simulink model "Wind"  (R2024b)
settings: Solver=ode23t  StartTime=0.0  StopTime=120  RelTol=1e-3
settings Model: Creator=Ioannis Vourkas  LastModifiedBy=HP

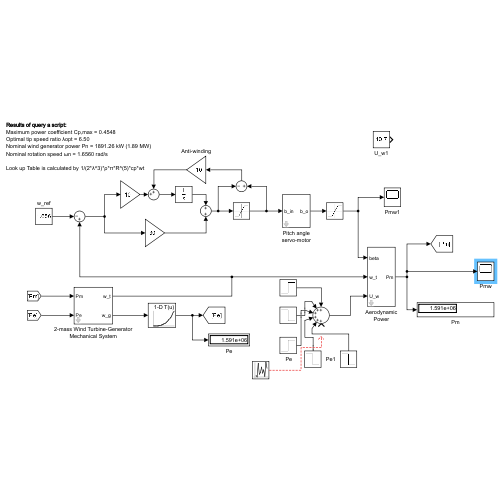
[thumbnail: Simulink's stored preview of the top-level diagram]
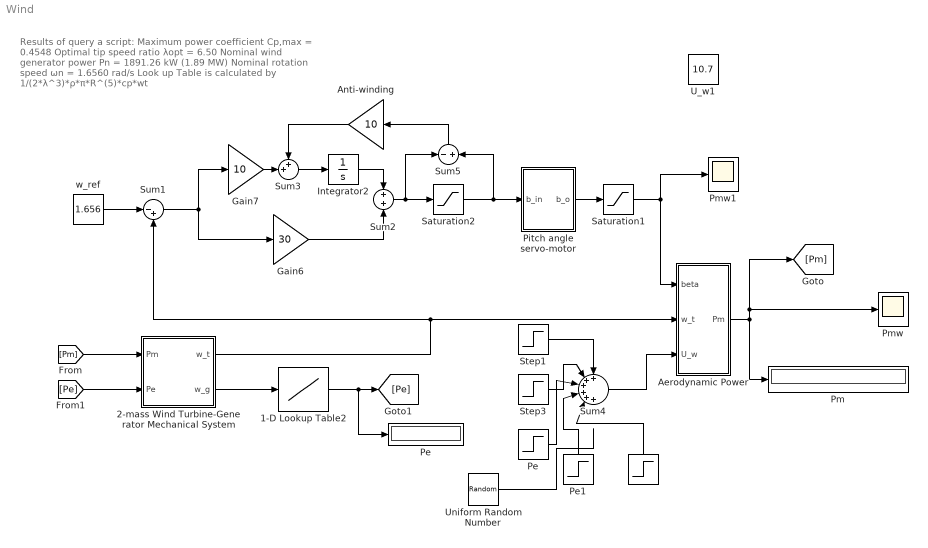
== system Wind ==
  note: Results of query a script:
      | Maximum power coefficient Cp,max = 0.4548
      | Optimal tip speed ratio λopt = 6.50
      | Nominal wind generator power Pn = 1891.26 kW (1.89 MW)
      | Nominal rotation speed ωn = 1.6560 rad/s
      |
      | Look up Table is calculated by 1/(2*λ^3)*ρ*π*R^(5)*cp*wt
  " " : Step  Time=35  After=-0.2  SampleTime=0
  " Pe" : Step  Time=20  After=0.45  SampleTime=0
  " Pe1" : Step  Time=25  After=-0.65  SampleTime=0
  1-D Lookup Table2 : Lookup_n-D  NumberOfTableDimensions=1  BreakpointsForDimension1=[0:0.05:1.656]  Table=416.257e3*[0:0.05:1.656].^3  InternalRulePriority=Speed  RndMeth=Simplest
  2-mass Wind Turbine-Generator Mechanical System : Subsystem  mask{K=15e6, D=5e6, Jt=8e6, Jn=100, w_init=1.65, w_inig=1.65}
      mask prompts: K "Elasticity"; D "Damping"; Jt "Turb Moment of Inertia"; Jn "Gen Moment of Inertia"; w_init "Initial turb w"; w_inig "Initial gen w"
  Aerodynamic Power : Subsystem  mask{R=42, ro=1.225, z=[0.0045, 0.0290], c=[0.22, 116.00, 0.20, 0.00, 5.00, 12.20]}
      mask prompts: R "Radius"; ro "Air density"; z "Z parameters"; c "C parameters"
  Anti-winding : Gain  Gain=10
  Gain6 : Gain  Gain=30
  Gain7 : Gain  Gain=10
  Integrator2 : Integrator
  Pe : Display
  Pitch angle servo-motor : Subsystem  mask{Tpam=0.2}
      mask prompts: Tpam "Pitch angle motor"
  Pm : Display
  Pmw : Scope
  Pmw1 : Scope
  Saturation1 : Saturate  UpperLimit=90  LowerLimit=0
  Saturation2 : Saturate  UpperLimit=90  LowerLimit=0
  Step1 : Step  Time=7  Before=10.7  After=11  SampleTime=0
  Step3 : Step  Time=13  Before=0.10  After=-0.5  SampleTime=0
  Sum1 : Sum  Inputs=|-+
  Sum2 : Sum  Inputs=+|+
  Sum3 : Sum  Inputs=++|
  Sum4 : Sum  Inputs=++++++
  Sum5 : Sum  Inputs=-|+
  U_w1 : Constant  Value=10.7
  Uniform Random Number : UniformRandomNumber  Minimum=1.3  Maximum=3.3  SampleTime=0.1
  w_ref : Constant  Value=1.656
  wires:
  Gain6/1 -> Sum2/2
  Integrator2/1 -> Sum2/1
  Gain7/1 -> Sum3/2
  Saturation1/1 -> Aerodynamic Power/1(beta), Pmw1/1
  Sum5/1 -> Anti-winding/1
  Anti-winding/1 -> Sum3/1
  Sum3/1 -> Integrator2/1
  Saturation2/1 -> Pitch angle servo-motor/1(b_in), Sum5/2
  Pitch angle servo-motor/1(b_o) -> Saturation1/1
  Sum2/1 -> Saturation2/1, Sum5/1
  Sum1/1 -> Gain6/1, Gain7/1
  w_ref/1 -> Sum1/1
  2-mass Wind Turbine-Generator Mechanical System/2(w_g) -> 1-D Lookup Table2/1
  2-mass Wind Turbine-Generator Mechanical System/1(w_t) -> Sum1/2, Aerodynamic Power/2(w_t)
  [Pe] -> 2-mass Wind Turbine-Generator Mechanical System/2(Pe)
  [Pm] -> 2-mass Wind Turbine-Generator Mechanical System/1(Pm)
  1-D Lookup Table2/1 -> Pe/1, [Pe]
  Aerodynamic Power/1(Pm) -> Pmw/1, [Pm], Pm/1
  Step3/1 -> Sum4/2
  " Pe"/1 -> Sum4/3
  Step1/1 -> Sum4/1
  " Pe1"/1 -> Sum4/4
  " "/1 -> Sum4/5
  Sum4/1 -> Aerodynamic Power/3(U_w)
  Uniform Random Number/1 -> ?

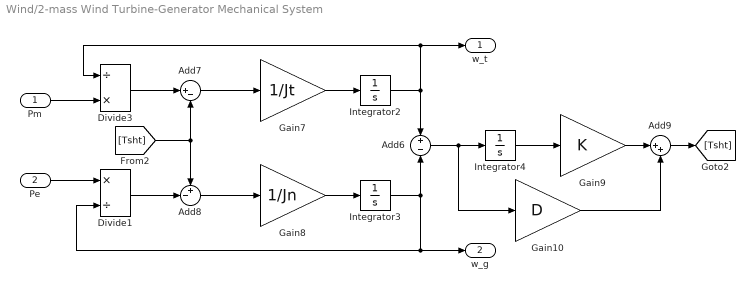
== system Wind/2-mass Wind Turbine-Generator Mechanical System ==
  Pm : Inport
  Pe : Inport  Port=2
  Add6 : Sum  Inputs=+|-
  Add7 : Sum  Inputs=|+-
  Add8 : Sum  Inputs=+-|
  Add9 : Sum  Inputs=|++
  Divide1 : Product  Inputs=*/
  Divide3 : Product  Inputs=/*
  Gain10 : Gain  Gain=D
  Gain7 : Gain  Gain=1/Jt
  Gain8 : Gain  Gain=1/Jn
  Gain9 : Gain  Gain=K
  Integrator2 : Integrator  InitialCondition=w_init
  Integrator3 : Integrator  InitialCondition=w_inig
  Integrator4 : Integrator  InitialCondition=0.35
  w_t : Outport
  w_g : Outport  Port=2
  wires:
  Pm/1 -> Divide3/2
  Pe/1 -> Divide1/1
  Add7/1 -> Gain7/1
  Add8/1 -> Gain8/1
  Gain9/1 -> Add9/1
  Divide3/1 -> Add7/1
  [Tsht] -> Add7/2, Add8/1
  Gain10/1 -> Add9/2
  Divide1/1 -> Add8/2
  Integrator4/1 -> Gain9/1
  Integrator3/1 -> Add6/2, w_g/1, Divide1/2
  Add6/1 -> Integrator4/1, Gain10/1
  Gain7/1 -> Integrator2/1
  Integrator2/1 -> w_t/1, Divide3/1, Add6/1
  Gain8/1 -> Integrator3/1
  Add9/1 -> [Tsht]

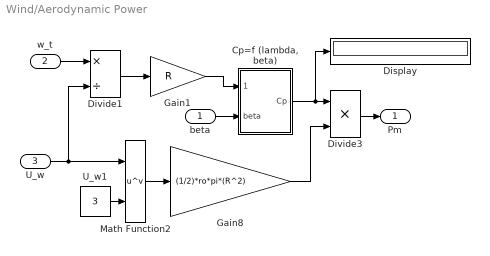
== system Wind/Aerodynamic Power ==
  beta : Inport
  w_t : Inport  Port=2
  U_w : Inport  Port=3
  "Cp=f (lambda, beta)" : Subsystem
  Display : Display
  Divide1 : Product  Inputs=*/
  Divide3 : Product  Inputs=**
  Gain1 : Gain  Gain=R
  Gain8 : Gain  Gain=(1/2)*ro*pi*(R^2)
  Math Function2 : Math  Operator=pow
  U_w1 : Constant  Value=3
  Pm : Outport
  wires:
  Gain1/1 -> "Cp=f (lambda, beta)"/1(lambda)
  Divide1/1 -> Gain1/1
  w_t/1 -> Divide1/1
  beta/1 -> "Cp=f (lambda, beta)"/2(beta)
  "Cp=f (lambda, beta)"/1(Cp) -> Divide3/1, Display/1
  Gain8/1 -> Divide3/2
  U_w1/1 -> Math Function2/2
  Divide3/1 -> Pm/1
  Math Function2/1 -> Gain8/1
  U_w/1 -> Math Function2/1, Divide1/2

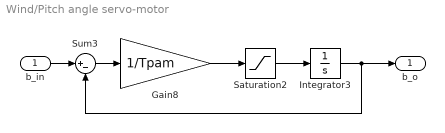
== system Wind/Pitch angle servo-motor ==
  b_in : Inport
  Gain8 : Gain  Gain=1/Tpam
  Integrator3 : Integrator
  Saturation2 : Saturate  UpperLimit=8  LowerLimit=-8
  Sum3 : Sum  Inputs=|+-
  b_o : Outport
  wires:
  Saturation2/1 -> Integrator3/1
  Integrator3/1 -> Sum3/2, b_o/1
  Gain8/1 -> Saturation2/1
  b_in/1 -> Sum3/1
  Sum3/1 -> Gain8/1

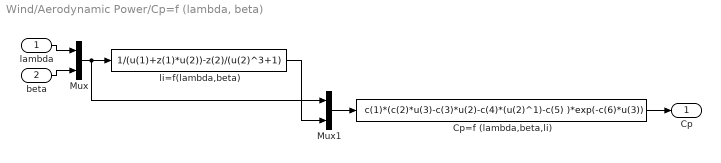
== system Wind/Aerodynamic Power/Cp=f (lambda, beta) ==
  lambda : Inport
  beta : Inport  Port=2
  Cp=f (lambda,beta,li) : Fcn  Expr=c(1)*(c(2)*u(3)-c(3)*u(2)-c(4)*(u(2)^1)-c(5) )*exp(-c(6)*u(3))  SampleTime=0
  Mux : Mux  Inputs=2
  Mux1 : Mux  Inputs=2
  li=f(lambda,beta) : Fcn  Expr=1/(u(1)+z(1)*u(2))-z(2)/(u(2)^3+1)  SampleTime=0
  Cp : Outport
  wires:
  Mux/1 -> li=f(lambda,beta)/1, Mux1/1
  Mux1/1 -> Cp=f (lambda,beta,li)/1
  li=f(lambda,beta)/1 -> Mux1/2
  lambda/1 -> Mux/1
  beta/1 -> Mux/2
  Cp=f (lambda,beta,li)/1 -> Cp/1
